simulink model "CompleteV1"  (R2024b)
settings: Solver=VariableStepAuto  StartTime=0.0  StopTime=inf  RelTol=1e-3
PreLoadFcn:
  | load("matlab.mat")
values from neighbouring files (symbols this model uses):
  BatteryOutput = 30    [matlab.mat]
undefined symbols (not defined in the file or in its folder): battery_soc, bay1_occupied, bay1_percentage, bay2_occupied, bay2_percentage, bay3_occupied, bay3_percentage, bay4_occupied, bay4_percentage, GridPeak, PVOutput
settings Model: PacingRate=10  Creator=bryan  LastModifiedBy=jason
settings DebuggingCC: UnderSpecifiedDimensionMsg=warning

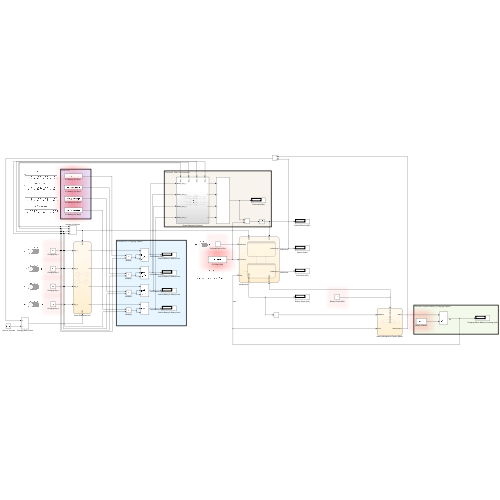
[thumbnail: Simulink's stored preview of the top-level diagram]
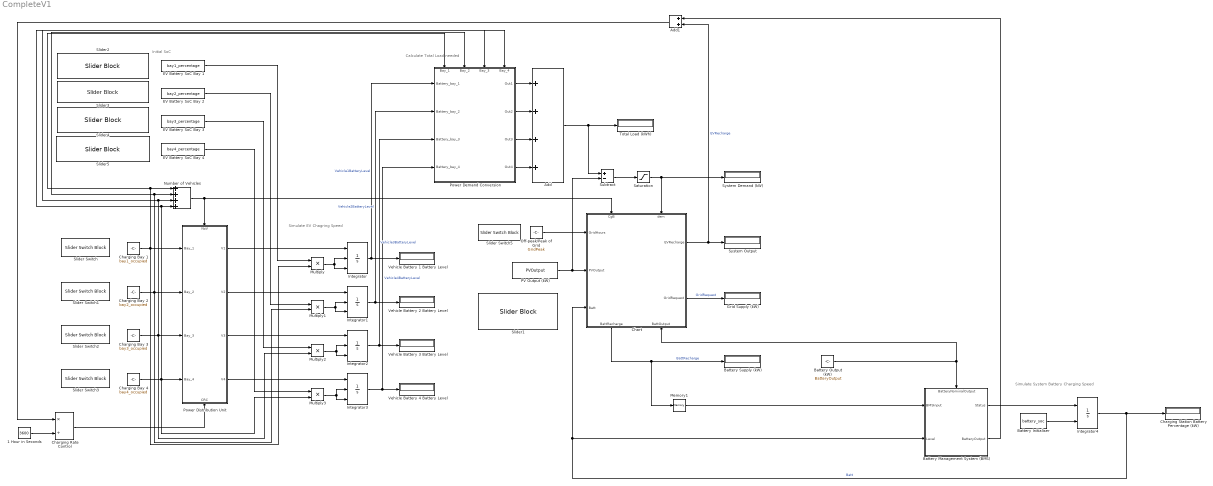
== system CompleteV1 ==
  note: Simulate System Battery Charging Speed
  note: Calculate Total Load needed
  note: Initial SoC
  note: Simulate EV Chagring Speed
  1 Hour in Seconds : Constant  Value=3600  OutDataTypeStr=int64
  Add : Sum  Inputs=++++
  Add1 : Sum
  Battery Initialiser : Constant  Value=battery_soc  OutDataTypeStr=double
  Battery Management System (BMS) : Stateflow chart  TreatAsAtomicUnit=on
      settings: PortSchema="{\"entries\":[{\"content\":{\"sides\":[{\"content\":{\"connectorIds\":[\"In2\",\"In3\"]},\"type\":\"ConnectorPlacement.EquallySpacedRectSide\",\"uuid\":\"9c5b3be8-4af2-4cee-ab11-9c77fe7daf26\"},{\"content\":{\"connectorIds\":[\"Out1\",\"Out2\"],\"side\":\"RIGHT\"},\"type\":\"ConnectorPlacement.EquallySpacedRectSide\",\"uuid\":\"cf6012c3-a30d-4793-b655-5b6bd2e00d27\"},{\"content\":{\"connectorIds\":[\"In1\"],\"side\":\"TOP\"},\"type\":\"ConnectorPlacement.EquallySpacedRectSide\",\"uuid\":\"7e2c1181-9fa3-4fe9-b0d9-b58d72dc862f\"}]},\"type\":\"ConnectorPlacement.EquallySpacedConnector\",\"uuid\":\"0afc5c89-b7cb-47f4-8376-469aa9da6e28\"}],\"packageUris\":[\"http://schema.mathworks.com/mf0/Connector/R2020b\"],\"version\":\"1.0\"}"
  Battery Output (kW) : Constant  Value=BatteryOutput
  Battery Supply (kW) : Display
  Charging Bay 1 : Constant  Value=bay1_occupied
  Charging Bay 2 : Constant  Value=bay2_occupied
  Charging Bay 3 : Constant  Value=bay3_occupied
  Charging Bay 4 : Constant  Value=bay4_occupied
  Charging Rate Control : Product  Inputs=*/
  Charging Station Battery Percentage (kW) : Display
  Chart : Stateflow chart  TreatAsAtomicUnit=on
      settings: PortSchema="{\"entries\":[{\"content\":{\"sides\":[{\"content\":{\"connectorIds\":[\"In4\",\"In5\",\"In6\"]},\"type\":\"ConnectorPlacement.EquallySpacedRectSide\",\"uuid\":\"3a5e50b6-7fb8-4c7e-aeea-20ecc3781894\"},{\"content\":{\"connectorIds\":[\"Out1\",\"Out2\"],\"side\":\"RIGHT\"},\"type\":\"ConnectorPlacement.EquallySpacedRectSide\",\"uuid\":\"e32e4170-0682-449c-9f07-66a5237a25e1\"},{\"content\":{\"connectorIds\":[\"In2\",\"In3\"],\"side\":\"TOP\"},\"type\":\"ConnectorPlacement.EquallySpacedRectSide\",\"uuid\":\"1da73483-e505-4e10-a78a-510adcca56f5\"},{\"content\":{\"connectorIds\":[\"Out3\",\"In1\"],\"side\":\"BOTTOM\"},\"type\":\"ConnectorPlacement.EquallySpacedRectSide\",\"uuid\":\"8ed36f85-eccb-4c99-bc71-cbd478a0e121\"}]},\"type\":\"ConnectorPlacement.EquallySpacedConnector\",\"uuid\":\"ab94fc83-fff0-4c66-b94d-14496d23ea6d\"}],\"packageUris\":[\"http://schema.mathworks.com/mf0/Connector/R2020b\"],\"version\":\"1.0\"}"
  EV Battery SoC Bay 1 : Constant  Value=bay1_percentage
  EV Battery SoC Bay 2 : Constant  Value=bay2_percentage
  EV Battery SoC Bay 3 : Constant  Value=bay3_percentage
  EV Battery SoC Bay 4 : Constant  Value=bay4_percentage
  Grid Supply (kW) : Display
  Integrator{,1..3} (4 alike) : Integrator  ExternalReset=either  InitialConditionSource=external  LimitOutput=on  UpperSaturationLimit=100  LowerSaturationLimit=0
  Integrator4 : Integrator  InitialConditionSource=external  LimitOutput=on  UpperSaturationLimit=100  LowerSaturationLimit=0
  Memory1 : Memory
  Multiply{,1..3} (4 alike) : Product  Inputs=**  OutDataTypeStr=double
  Number of Vehicles : Sum  Inputs=++++
  Off-peak/Peak of Grid : Constant  Value=GridPeak
  PV Output (kW) : Constant  Value=PVOutput
  Power Demand Conversion : Subsystem
      settings: PortSchema="{\"entries\":[{\"content\":{\"sides\":[{\"content\":{\"connectorIds\":[\"In1\",\"In2\",\"In3\",\"In4\"]},\"type\":\"ConnectorPlacement.EquallySpacedRectSide\",\"uuid\":\"042383c7-0e25-4693-9dd5-53273cd7df31\"},{\"content\":{\"connectorIds\":[\"Out1\",\"Out2\",\"Out3\",\"Out4\"],\"side\":\"RIGHT\"},\"type\":\"ConnectorPlacement.EquallySpacedRectSide\",\"uuid\":\"fa1d4f07-48f9-4d9b-82ba-6123af8bb58a\"},{\"content\":{\"connectorIds\":[\"In5\",\"In6\",\"In7\",\"In8\"],\"side\":\"TOP\"},\"type\":\"ConnectorPlacement.EquallySpacedRectSide\",\"uuid\":\"7c7c426f-e74b-4085-9c9e-1c7ce07c3bb9\"}]},\"type\":\"ConnectorPlacement.EquallySpacedConnector\",\"uuid\":\"cabe412c-a874-41d9-9fd4-692999f8238e\"}],\"packageUris\":[\"http://schema.mathworks.com/mf0/Connector/R2020b\"],\"version\":\"1.0\"}"
  Power Distribution Unit : Stateflow chart  TreatAsAtomicUnit=on
      settings: PortSchema="{\"entries\":[{\"content\":{\"sides\":[{\"content\":{\"connectorIds\":[\"In4\",\"In3\",\"In5\",\"In6\"]},\"type\":\"ConnectorPlacement.EquallySpacedRectSide\",\"uuid\":\"0f19e66f-83f1-44cb-8300-f799a0bdfb7f\"},{\"content\":{\"connectorIds\":[\"Out1\",\"Out2\",\"Out3\",\"Out4\"],\"side\":\"RIGHT\"},\"type\":\"ConnectorPlacement.EquallySpacedRectSide\",\"uuid\":\"6183555e-073a-46fe-9580-b02916d76341\"},{\"content\":{\"connectorIds\":[\"In1\"],\"side\":\"TOP\"},\"type\":\"ConnectorPlacement.EquallySpacedRectSide\",\"uuid\":\"01ca3085-7739-4a8d-b30f-46afdaf5bcd0\"},{\"content\":{\"connectorIds\":[\"In2\"],\"side\":\"BOTTOM\"},\"type\":\"ConnectorPlacement.EquallySpacedRectSide\",\"uuid\":\"e0a765b3-dcfc-42f9-8203-5cfe8b19df95\"}]},\"type\":\"ConnectorPlacement.EquallySpacedConnector\",\"uuid\":\"027b3a4e-d769-48e5-b718-313814246142\"}],\"packageUris\":[\"http://schema.mathworks.com/mf0/Connector/R2020b\"],\"version\":\"1.0\"}"
  Saturation : Saturate  UpperLimit=+inf  LowerLimit=0
  Slider Switch{,1..3,5} (5 alike) : SliderSwitchBlock
      settings: Values={{'Off', 'On'}, [0 1]}
  Slider{1..5} (5 alike) : SliderBlock
  Subtract : Sum  Inputs=+-
  System Demand (kW) : Display
  System Output : Display
  Total Load (kWh) : Display
      settings: Decimation=2
  Vehicle Battery 1 Battery Level : Display
  Vehicle Battery 2 Battery Level : Display
  Vehicle Battery 3 Battery Level : Display
  Vehicle Battery 4 Battery Level : Display
  wires:
  Power Distribution Unit/1(V1) -> Integrator/1
  Number of Vehicles/1 -> Power Distribution Unit/1(NoV), Chart/2(CgB)
  EV Battery SoC Bay 3/1 -> Multiply2/1
  Integrator/1 -> Vehicle Battery 1 Battery Level/1, Power Demand Conversion/1(Battery_bay_1)  "Vehicle1BatteryLevel"
  Charging Bay 4/1 -> Multiply3/2, Power Demand Conversion/8(Bay_4), Number of Vehicles/4, Power Distribution Unit/6(Bay_4)
  Charging Rate Control/1 -> Power Distribution Unit/2(CRC)
  Integrator1/1 -> Power Demand Conversion/2(Battery_bay_2), Vehicle Battery 2 Battery Level/1  "Vehicle2BatteryLevel"
  EV Battery SoC Bay 1/1 -> Multiply/1
  Add/1 -> Subtract/1, Total Load (kWh)/1
  Integrator2/1 -> Power Demand Conversion/3(Battery_bay_3), Vehicle Battery 3 Battery Level/1  "Vehicle3BatteryLevel"
  EV Battery SoC Bay 4/1 -> Multiply3/1
  Power Demand Conversion/2(Out2) -> Add/2
  Battery Management System (BMS)/2(BatteryOutput) -> Add1/1
  Power Demand Conversion/3(Out3) -> Add/3
  Power Distribution Unit/4(V4) -> Integrator3/1
  Memory1/1 -> Battery Management System (BMS)/2(BMSInput)
  Battery Management System (BMS)/1(Status) -> Integrator4/1
  Multiply/1 -> Integrator/2, Integrator/3
  PV Output (kW)/1 -> Subtract/2, Chart/5(PVOutput)
  Subtract/1 -> Saturation/1
  1 Hour in Seconds/1 -> Charging Rate Control/2
  Charging Bay 3/1 -> Multiply2/2, Power Demand Conversion/7(Bay_3), Number of Vehicles/3, Power Distribution Unit/5(Bay_3)
  Chart/1(EVRecharge) -> Add1/2, System Output/1  "EVRecharge"
  Power Distribution Unit/3(V3) -> Integrator2/1
  Integrator3/1 -> Power Demand Conversion/4(Battery_bay_4), Vehicle Battery 4 Battery Level/1  "Vehicle4BatteryLevel"
  Battery Initialiser/1 -> Integrator4/2
  Charging Bay 2/1 -> Power Demand Conversion/6(Bay_2), Number of Vehicles/2, Multiply1/2, Power Distribution Unit/3(Bay_2)
  Power Distribution Unit/2(V2) -> Integrator1/1
  Multiply2/1 -> Integrator2/2, Integrator2/3
  Battery Output (kW)/1 -> Battery Management System (BMS)/1(BatteryNominalOutput), Chart/1(BattOutput)
  Power Demand Conversion/4(Out4) -> Add/4
  Multiply3/1 -> Integrator3/2, Integrator3/3
  Chart/2(GridRequest) -> Grid Supply (kW)/1  "GridRequest"
  EV Battery SoC Bay 2/1 -> Multiply1/1
  Charging Bay 1/1 -> Power Demand Conversion/5(Bay_1), Number of Vehicles/1, Multiply/2, Power Distribution Unit/4(Bay_1)
  Saturation/1 -> System Demand (kW)/1, Chart/3(dem)
  Power Demand Conversion/1(Out1) -> Add/1
  Integrator4/1 -> Chart/6(Batt), Battery Management System (BMS)/3(Level), Charging Station Battery Percentage (kW)/1  "Batt"
  Off-peak/Peak of Grid/1 -> Chart/4(GridHours)
  Multiply1/1 -> Integrator1/2, Integrator1/3
  Chart/3(BattRecharge) -> Battery Supply (kW)/1, Memory1/1  "BattRecharge"
  Add1/1 -> Charging Rate Control/1

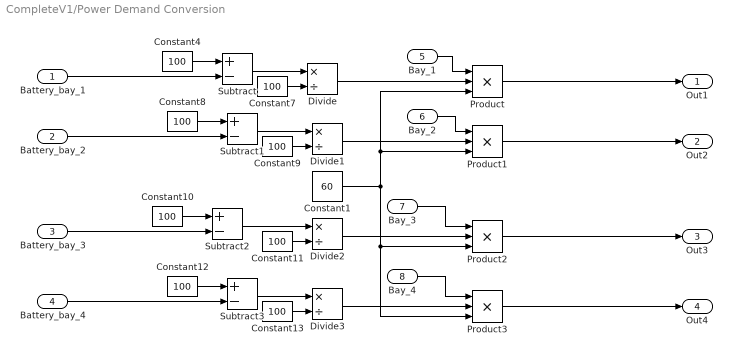
== system CompleteV1/Power Demand Conversion ==
  Battery_bay_1 : Inport
  Battery_bay_2 : Inport  Port=2
  Battery_bay_3 : Inport  Port=3
  Battery_bay_4 : Inport  Port=4
  Bay_1 : Inport  Port=5
  Bay_2 : Inport  Port=6
  Bay_3 : Inport  Port=7
  Bay_4 : Inport  Port=8
  Constant1 : Constant  Value=60
  Constant{4,7..13} (8 alike) : Constant  Value=100
  Divide{,1..3} (4 alike) : Product  Inputs=*/
  Product{,1..3} (4 alike) : Product  Inputs=3
  Subtract{,1..3} (4 alike) : Sum  Inputs=+-
  Out1 : Outport
  Out2 : Outport  Port=2
  Out3 : Outport  Port=3
  Out4 : Outport  Port=4
  wires:
  Constant4/1 -> Subtract/1
  Constant9/1 -> Divide1/2
  Battery_bay_2/1 -> Subtract1/2
  Subtract/1 -> Divide/1
  Subtract3/1 -> Divide3/1
  Constant11/1 -> Divide2/2
  Subtract1/1 -> Divide1/1
  Constant13/1 -> Divide3/2
  Constant8/1 -> Subtract1/1
  Constant12/1 -> Subtract3/1
  Constant7/1 -> Divide/2
  Battery_bay_1/1 -> Subtract/2
  Constant10/1 -> Subtract2/1
  Subtract2/1 -> Divide2/1
  Battery_bay_4/1 -> Subtract3/2
  Battery_bay_3/1 -> Subtract2/2
  Divide/1 -> Product/2
  Divide1/1 -> Product1/2
  Divide2/1 -> Product2/2
  Constant1/1 -> Product3/3, Product2/3, Product/3, Product1/3
  Divide3/1 -> Product3/2
  Product/1 -> Out1/1
  Product1/1 -> Out2/1
  Product2/1 -> Out3/1
  Product3/1 -> Out4/1
  Bay_1/1 -> Product/1
  Bay_2/1 -> Product1/1
  Bay_3/1 -> Product2/1
  Bay_4/1 -> Product3/1

== stateflow chart CompleteV1/Power Distribution Unit ==
  state No1
    V1 = Bay_1 * CRC;
    V2 = Bay_2 * CRC;
    V3 = Bay_3 * CRC;
    V4 = Bay_4 * CRC;
  state No2
    V1 = Bay_1 * CRC/2;
    V2 = Bay_2 * CRC/2;
    V3 = Bay_3 * CRC/2;
    V4 = Bay_4 * CRC/2;
  state No4
    V1 = Bay_1 * CRC/4;
    V2 = Bay_2 * CRC/4;
    V3 = Bay_3 * CRC/4;
    V4 = Bay_4 * CRC/4;
  state No3
    V1 = Bay_1 * CRC/3;
    V2 = Bay_2 * CRC/3;
    V3 = Bay_3 * CRC/3;
    V4 = Bay_4 * CRC/3;
  (default) -> No1
  No1 -> No2 [order 1] : [NoV > 1]
  No2 -> No1 [order 1] : [NoV == 1]
  No4 -> No1 [order 2] : [NoV == 1]
  No1 -> No4 [order 2] : [NoV == 4]
  No2 -> No3 [order 2] : [NoV > 2]
  No3 -> No2 [order 1] : [NoV < 3]
  No4 -> No3 [order 1] : [NoV < 4]
  No3 -> No4 [order 2] : [NoV == 4]
  data: NoV input; CRC input; Bay_2 input; Bay_1 input; Bay_3 input; Bay_4 input; V1 output; V2 output; V3 output; V4 output

== stateflow chart CompleteV1/Chart ==
  state Offpeak
    state Car01
      EVRecharge = (60*CgB);
      BattRecharge  = 60;
      GridRequest = EVRecharge + BattRecharge;
    state Idle
    state CarOver1
      EVRecharge = (60*CgB);
      BattRecharge = 0;
      GridRequest = EVRecharge + BattRecharge;
    (default) -> Offpeak.Idle
    Offpeak.Idle -> Car01 [order 2] : [CgB < 2]
    Car01 -> Offpeak.Idle : [CgB > 1 || Batt > 100]
    Offpeak.Idle -> Offpeak.CarOver1 [order 1] : [CgB > 1]
    Offpeak.CarOver1 -> Offpeak.Idle : [CgB < 2]
  state Peak
    state Car0
      EVRecharge = (60*CgB);
      BattRecharge = PVOutput;
      GridRequest = 0;
    state CarOver1
      EVRecharge = (60*CgB);
      BattRecharge = (-1)*(BattOutput);
      GridRequest = EVRecharge - (PVOutput + BattOutput);
    state Idle
    state CarOver1andBattLow
      EVRecharge = (60*CgB);
      BattRecharge = 0;
      GridRequest = EVRecharge - PVOutput;
    (default) -> Peak.Idle
    Car0 -> Peak.Idle : [CgB > 0 || Batt > 100]
    Peak.Idle -> Peak.CarOver1 [order 2] : [CgB  > 0]
    Peak.Idle -> Car0 [order 3] : [CgB == 0 && Batt < 95]
    Peak.CarOver1 -> Peak.Idle : [CgB > 1 || Batt > 100]
    Peak.Idle -> CarOver1andBattLow [order 1] : [CgB > 0 && Batt < 10]
    CarOver1andBattLow -> Peak.Idle : [CgB < 1]
  Offpeak -> Peak : [GridHours == 1]
  Peak -> Offpeak : [GridHours == 0]
  (default) -> Peak
  data: BattOutput input; CgB input; dem input; EVRecharge output =0; GridRequest output; GridHours input; PVOutput input double; Batt input; BattRecharge output

== stateflow chart CompleteV1/Battery Management System (BMS) ==
  note: Status
      | 0 - Idle
      | 1 - Charging
      | 2 - Discharge
  state Charging
    Status = (BMSInput/3600);
    BatteryOutput=0;
  state Discharging
    Status = ((-1)*BatteryNominalOutput)/3600 ;
    BatteryOutput=30;
  state Idle
    Status = 0;
  Discharging -> Charging [order 2] : [BMSInput > 1]
  Charging -> Discharging [order 2] : [BMSInput < 0]
  Charging -> Idle [order 3] : [BMSInput == 0]
  Discharging -> Idle [order 3] : [BMSInput == 0]
  (default) -> Discharging
  Discharging -> Idle [order 1] : [Level <= 20]
  Charging -> Idle [order 1] : [Level >= 95]
  Idle -> Charging [order 2] : [BMSInput > 1 && Level < 95]
  Idle -> Discharging [order 1] : [BMSInput < 0 && Level > 10]
  data: BatteryNominalOutput input; Status output; BMSInput input; Level input; BatteryOutput output
